simulink library "EMTAT_Libraries_PowerFlow_Lib_PFSys_GenericInverter_TMATS"  (R2019b)
settings: Solver=ode45  StartTime=0.0  StopTime=10.0  RelTol=1e-3  EnableMultiTasking=on
libraries: simulink x1
Description:
  | Thomas Modules
settings Model: Creator=jwchapm2  LastModifiedBy=sbianco1
settings DataIOCC: LimitDataPoints=on  SaveFormat=Array  ReturnWorkspaceOutputs=off
settings OptimizationCC: ExpressionDepthLimit=2147483647  LifeSpan=inf
settings DebuggingCC: UnderspecifiedInitializationDetection=Classic  MergeDetectMultiDrivingBlocksExec=none  SolverPrmCheckMsg=warning  StateNameClashWarn=warning  SFUnexpectedBacktrackingDiag=warning  SFNoUnconditionalDefaultTransitionDiag=warning  SFExecutionAtInitializationDiag=none  ArithmeticOperatorsInVariantConditions=warning
settings HardwareCC: ProdBitPerPointer=32  ProdBitPerSizeT=32  ProdBitPerPtrDiffT=32  ProdLargestAtomicFloat=None  ProdIntDivRoundTo=Undefined  ProdEndianess=Unspecified  ProdWordSize=32  ProdHWDeviceType=32-bit Generic
settings ModelReferenceCC: PropagateSignalLabelsOutOfModel=off
settings SFSimCC: SimUseLocalCustomCode=off  CustomCodeUndefinedFunction=UseInterfaceOnly
settings RTWCC: RTWUseLocalCustomCode=off
settings CodeAppCC: StateflowObjectComments=on
settings GRTTargetCC: TargetLangStandard=C89/C90 (ANSI)  GeneratePreprocessorConditionals=Disable all
settings ConfigComp: CovMetricSettings=dw  CovHtmlReporting=on  CovSaveCumulativeToWorkspaceVar=on  CovSaveSingleToWorkspaceVar=on  CovExternalEMLEnable=off

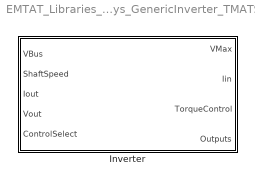
== system EMTAT_Libraries_PowerFlow_Lib_PFSys_GenericInverter_TMATS ==
  "Inverter " : Subsystem  mask(Inverter){Hz_to_V_M=22, X_C_VoltageVec_M=[0.0 0.1 1.0], Y_C_CurrentVec_M=[0.0 0.1 1.0], T_C_EffArray_M=[0.5 0.5 0.5; 0.5 1.0 1.0; 0.5 1.0 1.0], Pdis_M=1, mode=Speed Control, P=0.61652, I=7.6146, D=0, Filt=100, Js=0.01, bs=0, tau=0.1, SetAmp=2000}
      mask prompts: Hz_to_V_M "Hz_to_V_M - Voltage/Flux Constant"; X_C_VoltageVec_M "X_C_VoltageVec_M - Efficiency Table Voltage Vector (X-axis)(nx1), V"; Y_C_CurrentVec_M "Y_C_CurrentVec_M - Efficiency Table Current Vector (Y-axis)(mx1), A"; T_C_EffArray_M "T_C_EffArray_M - Efficiency Table Values (Eff = f(i, V)(nxm)"; Pdis_M "Pdis_M - Constant Power Leaked/Dissipated, W"; P "Kp - Proportional Gain"; I "Ki - Integral Gain"; D "Kd - Derivative Gain"; Filt "Filt - Filter Coefficient"; Js "Js - Shaft Inertia, lbf-ft-s^2"; bs "bs - Shaft Damping, lbf-ft-s"; tau "tau - Motor Response Time, s"; SetAmp "SetAmp - Design Setpoint, RPM"
      mask help:
      | This block represents a DC-to-AC inverter (for motor control). The block
      | produces an output voltage that scales with input frequency accoring to
      | the flux constant, Hz_to_V_M. The load is assumed to have no inductance,
      | and so we are assumed to operate with unity power factor. Converter
      | efficiency is specified via a lookup table that is a function of output
      | voltage and output current.
      mask TypeOptions mode: Speed Control | Torque Control
      mask Callback mode:
      | param_values = get_param(gcb,'MaskValues');
      | param_enable = get_param(gcb,'MaskEnables');
      | mode = param_values(6);
      | mode = mode{1};
      | if strcmp(mode,'Speed Control')
      |     param_enable(7) = {'on'}; %P
      |     param_enable(8) = {'on'}; %I
      |     param_enable(9) = {'on'}; %D
      |     param_enable(10) = {'on'}; %Filter
      |     param_enable(11) = {'on'}; %Inertia
      |     param_enable(12) = {'on'}; %Damping
      |     param_enable(13) = {'on'}; %Response
      |     param_enable(14) = {'on'}; %StepAmplitude
      |     set_param(gcb,'MaskEnables',param_enable)
      |     maskHandle = Simulink.Mask.get(gcb);
      |     buttonHandle = maskHandle.getDialogControl('iDesignButton');
      |     buttonHandle.Enabled = 'on';
      | elseif strcmp(mode,'Torque Control')
      |     param_enable(7) = {'off'}; %P
      |     param_enable(8) = {'off'}; %I
      |     param_enable(9) = {'off'}; %D
      |     param_enable(10) = {'off'}; %Filter
      |     param_enable(11) = {'off'}; %Inertia
      |     param_enable(12) = {'off'}; %Damping
      |     param_enable(13) = {'off'}; %Response
      |     param_enable(14) = {'off'}; %StepAmplitude
      |     set_param(gcb,'MaskEnables',param_enable)
      |     maskHandle = Simulink.Mask.get(gcb);
      |     buttonHandle = maskHandle.getDialogControl('iDesignButton');
      |     buttonHandle.Enabled = 'off';
      | end
      mask DialogControl Container6 Prompt: Parameters
      mask DialogControl Container8 Prompt: Inverter
      mask DialogControl Container9 Prompt: Controller
      mask DialogControl Container17 Prompt: iDesign
      mask DialogControl Container18 Prompt: Controller
      mask DialogControl SetAmp Tooltip: The magnitude of the step responce plotted after controller iDesign is ran. Use an average of your controller setpoint as your design setpoint.
      mask DialogControl iDesignButton Prompt: Run iDesign
      mask DialogControl iDesignButton Callback: run('run_iDesign_SpeedController')
      mask Display:
      | % Port labels and block information
      | 
      | port_label('output', 1, 'VMax');
      | port_label('output', 2, 'Iin');
      | port_label('output', 3, 'TorqueControl');
      | port_label('output', 4, 'Outputs');
      | 
      | port_label('input', 1, 'VBus');
      | port_label('input', 2, 'ShaftSpeed');
      | port_label('input', 3, 'Iout');
      | port_label('input', 4, 'Vout');
      | switch mode
      |     case 1
      |         fprintf('Inverter\nin\nSpeed Control')
      |         port_label('input', 5, 'SpeedSet');
      |     case 2
      |         fprintf('Inverter\nin\nTorque Control')
      |         port_label('input', 5, 'TorqueSet');
      | end

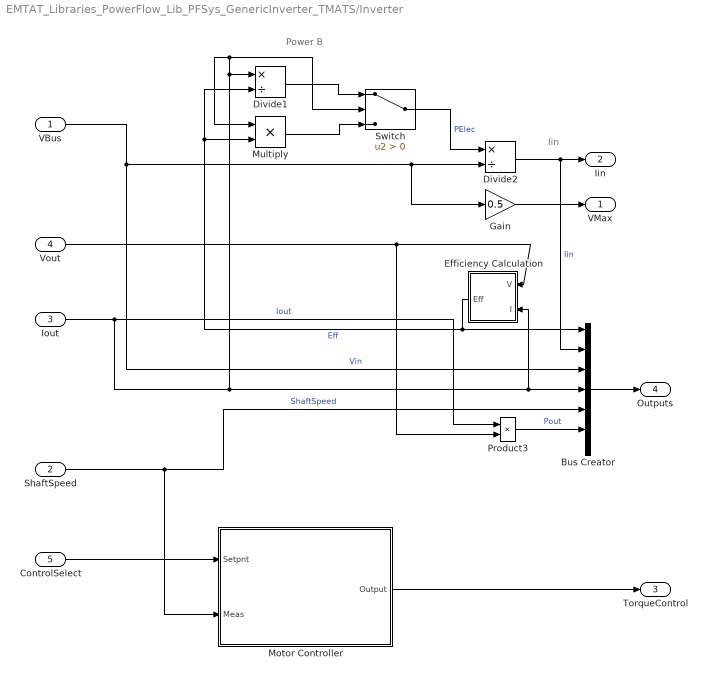
== system EMTAT_Libraries_PowerFlow_Lib_PFSys_GenericInverter_TMATS/Inverter  ==
  note: Iin
  note: Power B
  VBus : Inport
  "ShaftSpeed " : Inport  Port=2
  Iout : Inport  Port=3
  Vout : Inport  Port=4
  ControlSelect : Inport  Port=5
  Bus Creator : BusCreator  Inputs=7
  Divide1 : Product  Inputs=*/
  Divide2 : Product  Inputs=*/
  Efficiency Calculation : Subsystem
  Gain : Gain  Gain=0.5
  Motor Controller : Subsystem
  Multiply : Product
  Product3 : Product
  Switch : Switch  Criteria=u2 > Threshold
  VMax : Outport  VectorParamsAs1DForOutWhenUnconnected=off
  Iin : Outport  Port=2  VectorParamsAs1DForOutWhenUnconnected=off
  TorqueControl : Outport  Port=3
  Outputs : Outport  Port=4  VectorParamsAs1DForOutWhenUnconnected=off
  wires:
  Product3/1 -> Bus Creator/6  "Pout"
  Bus Creator/1 -> Outputs/1
  "ShaftSpeed "/1 -> Motor Controller/2(Meas), Bus Creator/5  "ShaftSpeed"
  VBus/1 -> Gain/1, Divide2/2, Bus Creator/3  "Vin"
  Iout/1 -> Product3/1, Bus Creator/4, Efficiency Calculation/2(I), Multiply/1, Switch/2, Divide1/1  "Iout"
  Gain/1 -> VMax/1
  Efficiency Calculation/1(Eff) -> Divide1/2, Multiply/2, Bus Creator/1  "Eff"
  Multiply/1 -> Switch/3
  Divide1/1 -> Switch/1
  Switch/1 -> Divide2/1  "PElec"
  Vout/1 -> Product3/2, Efficiency Calculation/1(V)
  Divide2/1 -> Bus Creator/2, Iin/1  "Iin"
  ControlSelect/1 -> Motor Controller/1(Setpnt)
  Motor Controller/1(" Output") -> TorqueControl/1

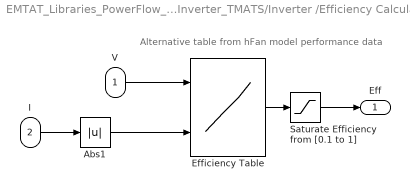
== system EMTAT_Libraries_PowerFlow_Lib_PFSys_GenericInverter_TMATS/Inverter /Efficiency Calculation ==
  note: Alternative table from hFan model performance data
  V : Inport
  I : Inport  Port=2
  Abs1 : Abs
  Efficiency Table : Lookup_n-D  BreakpointsForDimension1=X_C_VoltageVec_M  BreakpointsForDimension2=Y_C_CurrentVec_M  Table=T_C_EffArray_M  ExtrapMethod=Clip  InternalRulePriority=Speed  RndMeth=Simplest  InputSameDT=on
  Saturate Efficiency from [0.1 to 1] : Saturate  UpperLimit=1  LowerLimit=0.1
  Eff : Outport  VectorParamsAs1DForOutWhenUnconnected=off
  wires:
  Abs1/1 -> Efficiency Table/2
  Saturate Efficiency from [0.1 to 1]/1 -> Eff/1
  Efficiency Table/1 -> Saturate Efficiency from [0.1 to 1]/1
  I/1 -> Abs1/1
  V/1 -> Efficiency Table/1

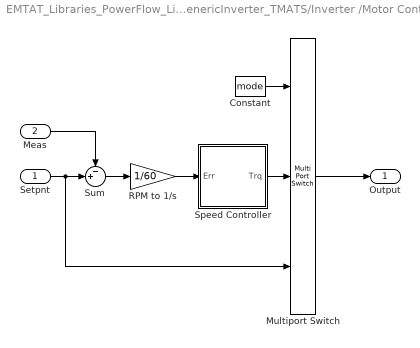
== system EMTAT_Libraries_PowerFlow_Lib_PFSys_GenericInverter_TMATS/Inverter /Motor Controller ==
  Setpnt : Inport
  Meas : Inport  Port=2
  Constant : Constant  Value=mode
  Multiport Switch : MultiPortSwitch  Inputs=2
  RPM to 1/s : Gain  Gain=1/60
  Speed Controller : Subsystem
  Sum : Sum  Inputs=-+|
  " Output" : Outport
  wires:
  Multiport Switch/1 -> " Output"/1
  Meas/1 -> Sum/1
  RPM to 1/s/1 -> Speed Controller/1(Err)
  Setpnt/1 -> Sum/2, Multiport Switch/3
  Speed Controller/1(Trq) -> Multiport Switch/2
  Sum/1 -> RPM to 1/s/1
  Constant/1 -> Multiport Switch/1

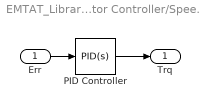
== system EMTAT_Libraries_PowerFlow_Lib_PFSys_GenericInverter_TMATS/Inverter /Motor Controller/Speed Controller ==
  Err : Inport
  PID Controller : simulink/Continuous/PID Controller  Controller=PID  Form=Parallel  TimeDomain=Continuous-time  SampleTime=-1  IntegratorMethod=Forward Euler  FilterMethod=Forward Euler  ControllerParametersSource=internal  P=P  I=I  D=D  UseFilter=on  N=Filt  TunerSelectOption=Transfer Function Based (PID Tuner App)  InitialConditionSource=internal  InitialConditionForIntegrator=0  InitialConditionForFilter=0  DifferentiatorICPrevScaledInput=0  ExternalReset=none  TrackingMode=off  Kt=1  LimitOutput=off  UpperSaturationLimit=inf  LowerSaturationLimit=-inf  LinearizeAsGain=on  AntiWindupMode=none  Kb=1  POutMin=[]  POutMax=[]  IOutMin=[]  IOutMax=[]  DOutMin=[]  DOutMax=[]  NOutMin=[]  NOutMax=[]  SumOutMin=[]  SumOutMax=[]  SaturationOutMin=[]  SaturationOutMax=[]  PParamMin=[]  PParamMax=[]  IParamMin=[]  IParamMax=[]  DParamMin=[]  DParamMax=[]  NParamMin=[]  NParamMax=[]  KbParamMin=[]  KbParamMax=[]  KtParamMin=[]  KtParamMax=[]  KbOutMin=[]  KbOutMax=[]  KtOutMin=[]  KtOutMax=[]  IntegratorOutMin=[]  IntegratorOutMax=[]  FilterOutMin=[]  FilterOutMax=[]  SumI1OutMin=[]  SumI1OutMax=[]  SumI2OutMin=[]  SumI2OutMax=[]  SumI3OutMin=[]  SumI3OutMax=[]  SumI4OutMin=[]  SumI4OutMax=[]  SumDOutMin=[]  SumDOutMax=[]  DifferentiatorOutMin=[]  DifferentiatorOutMax=[]  FilterDiffOutCoefMin=[]  FilterDiffOutCoefMax=[]  ReciprocalOutMin=[]  ReciprocalOutMax=[]  SumDenOutMin=[]  SumDenOutMax=[]  SumNumOutMin=[]  SumNumOutMax=[]  DivideOutMin=[]  DivideOutMax=[]  IntegratorContinuousStateAttributes=''  IntegratorStateMustResolveToSignalObject=off  IntegratorRTWStateStorageClass=Auto  FilterContinuousStateAttributes=''  FilterStateMustResolveToSignalObject=off  FilterRTWStateStorageClass=Auto  ParallelPVariant=InternalParameters  IdealPVariant=Disabled  IVariant=InternalParameters  DVariant=InternalParameters  IntegratorVariant=Continuous  SatVariant=Disabled  AWVariant=Passthrough  PCopyVariant=Disabled  TRVariant=Disabled  FdbkBlocksVariant=Forward  IdealPFdbkVariant=Disabled  SatFdbkVariant=Disabled  DerivativeFilterVariant=ContFilter  NVariant=InternalParameters  NCopyVariant=Disabled  FilterICVariant=InternalICsFilter  IntegratorICVariant=InternalICs  ExternalResetVariant=Disabled  TRSumVariant=Passthrough  SumFdbkVariant=Disabled  SumVariant=Sum_PID
  Trq : Outport
  wires:
  Err/1 -> PID Controller/1
  PID Controller/1 -> Trq/1
